simulink model "cruise_control_prop_error1"  (Simulink 7.8)
settings: Solver=FixedStepDiscrete  SolverMode=SingleTasking  StartTime=0.0  StopTime=50  FixedStep=0.01  RelTol=1e-3  AbsTol=1e-6
model workspace (MAT data in the model file):
  converter_data = [0  137.465208994  2.232; 0.1  137.065019157  2.075; 0.2  135.864449646  1.975; 0.3  135.664354728  1.846; 0.4  137.565256453  1.72; 0.5  140.366585312  1.564; 0.6  145.268910814  1.409; 0.7  152.872517717  1.254; 0.8  162.9773111  1.096; 0.81  164.27792807  1.08; 0.82  166.178829795  1.061; 0.83  167.979684062  1.043; 0.84  170.080680706  1.028; 0.85  172.781962105  1.012; 0.86  175.383196045  1.002; 0.87  179.585189333  1.002; 0.88  183.587087703  1.001; 0.89  189.890077635  0.998; 0.9  197.693779455  0.999; 0.92  215.902417037  1.001; 0.94  244.515990379  1.002]
  emap = [-40  -44  -49  -53  -57  -61  -65  -70  -74  -78  -82; 215  117  85  66  44  29  10  -2  -13  -22  -32; 245  208  178  148  122  104  85  66  48  33  18; 264  260  241  219  193  167  152  133  119  96  85; 264  279  282  275  260  238  223  208  189  171  152; 267  290  293  297  290  275  260  256  234  212  193; 267  297  305  305  305  301  293  282  267  249  226; 267  301  308  312  319  323  319  316  297  279  253; 267  301  312  319  327  327  327  327  312  293  267; 267  301  312  319  327  334  334  334  319  305  275]
  Iei = 0.0219914882836
  nevec = [800 1200 1600 2000 2400 2800 3200 3600 4000 4400 4800]
  p0 = 0.07934
  p1 = 0.07934
  thvec = [0; 20; 30; 40; 50; 60; 70; 80; 90; 100]
  vehicledata : num (value not decoded)
values from neighbouring files (symbols this model uses):
  cruise_ki = 0.01    [cruise_control_data.m]    (also in fxpdata_simulinkpackage.mat)
  cruise_kp = 0.02    [cruise_control_data.m]    (also in fxpdata_simulinkpackage.mat)
  speed_max = 300    [cruise_control_data.m]    (also in fxpdata_simulinkpackage.mat)
  speed_min = -50    [cruise_control_data.m]    (also in fxpdata_simulinkpackage.mat)
  target_max = 100    [cruise_control_data.m]    (also in fxpdata_simulinkpackage.mat)
  target_min = 30    [cruise_control_data.m]    (also in fxpdata_simulinkpackage.mat)
  throt_max = 100    [cruise_control_data.m]    (also in fxpdata_simulinkpackage.mat)
  throt_min = 0    [cruise_control_data.m]    (also in fxpdata_simulinkpackage.mat)
  vel_dec = 1    [cruise_control_data.m]    (also in fxpdata_simulinkpackage.mat)
  vel_inc = 1    [cruise_control_data.m]    (also in fxpdata_simulinkpackage.mat)
undefined symbols (not defined in the file or in its folder): DiscIntNeverNeededParam, sldvsubsys
libraries: sldvlib x29, propertySpecificationOperatorLib x8, simulink x1
settings Model: MinMaxOverflowLogging=MinMaxAndOverflow  FPTRunName=オーバーライドなし  Creator=The MathWorks Inc.  LastModifiedBy=itoy  CovMetricSettings=dcmtr  CovHTMLOptions=-aTS=1 -bRG=1 -bTC=1 -hTR=0 -nFC=0 -scm=1 -bcm=1 -xEv=0  ExtModeTrigMode=oneshot  ExtModeArmWhenConnect=off  ExtModeAutoUpdateStatusClock=off
settings DataIOCC: LimitDataPoints=off  SaveOutput=off  SaveTime=off  SignalLoggingName=mysig
settings OptimizationCC: InlineParams=on  UseIntDivNetSlope=on  UseFloatMulNetSlope=on  InlineInvariantSignals=on  EnhancedBackFolding=on  EfficientFloat2IntCast=on  LifeSpan=1
settings DebuggingCC: SignalInfNanChecking=error  SaveWithParameterizedLinksMsg=none  CheckExecutionContextPreStartOutputMsg=on  CheckExecutionContextRuntimeOutputMsg=on  SolverPrmCheckMsg=none  SingleTaskRateTransMsg=error  IntegerOverflowMsg=error  UniqueDataStoreMsg=error  BusObjectLabelMismatch=error  RootOutportRequireBusObject=error  AssertControl=DisableAll  StrictBusMsg=ErrorOnBusTreatedAsVector  BusNameAdapt=ErrorWithoutRepair  NonBusSignalsTreatedAsBus=error  LoggingUnavailableSignals=none
settings HardwareCC: ProdIntDivRoundTo=Zero  ProdEndianess=LittleEndian  ProdHWDeviceType=NEC->V850  TargetIntDivRoundTo=Zero  TargetEndianess=LittleEndian  TargetHWDeviceType=MATLAB Host
settings ModelReferenceCC: ModelReferenceNumInstancesAllowed=Single
settings SFSimCC: SFSimEcho=off  SimParseCustomCode=off
settings RTWCC: GenerateReport=on  ProcessScript=grt_make_rtw_hook  LaunchReport=on  IncludeERTFirstTime=on  RTWCompilerOptimization=On
settings ConfigComp: Description=Design Verifier Custom Configuration Component  DVMaxProcessTime=3000  DVDisplayUnsatisfiableObjectives=on  DVModelCoverageObjectives=MCDC  DVMaxTestCaseSteps=500  DVTestSuiteOptimization=LargeModel (Nonlinear Extended)

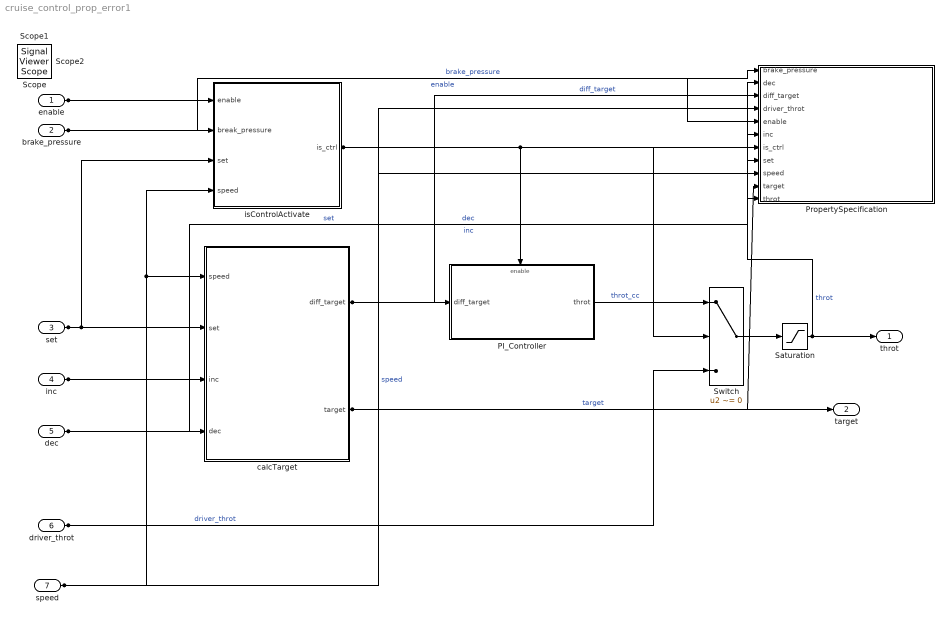
== system cruise_control_prop_error1 ==
  enable : Inport  PortDimensions=1  Interpolate=off
  brake_pressure : Inport  Port=2  PortDimensions=1  Interpolate=off
  set : Inport  Port=3  PortDimensions=1  Interpolate=off
  inc : Inport  Port=4  PortDimensions=1  Interpolate=off
  dec : Inport  Port=5  PortDimensions=1  Interpolate=off
  driver_throt : Inport  Port=6  PortDimensions=1  Interpolate=off
  speed : Inport  Port=7  PortDimensions=1  Interpolate=off
  PI_Controller : Subsystem
  PropertySpecification : Subsystem  Tag=VerificationSubsystem  DisableCoverage=on  LoadFcn=sldvsubsys('check')  TreatAsAtomicUnit=on  SimViewingDevice=on  mask(VerificationSubsystem){}
      mask help: aa
      mask init:
      | sldvsubsys('maskInit');
      settings: OpenFcn=PropertySpecificationUI('Block',gcb)
      settings: CopyFcn=|
      | sldvsubsys('copy');
      |  set_param(gcb,'LinkStatus','none')
      settings: PreSaveFcn=|
      | set_param(gcb,'SimViewingDevice','on');
      | sldvsubsys('check');
      mask Help: helpview(fullfile(docroot,'toolbox','sldv','sldv.map'),'verificationsubsystem')
      mask Display: image(imread('sldvicon_versubsys.png','BackGroundColor',[1 1 1]),'center');
  Saturation : Saturate  UpperLimit=throt_max  LowerLimit=throt_min  OutDataTypeStr=Inherit: Inherit via back propagation
      settings: AttributesFormatString=<UpperLimit = %<UpperLimit>>\n<LowerLimit = %<LowerLimit>>
  Switch : Switch  Criteria=u2 ~= 0  OutDataTypeStr=Inherit: Inherit via back propagation
      settings: AttributesFormatString=<Criteria=%<Criteria>>
  calcTarget : Subsystem
  isControlActivate : Subsystem
  throt : Outport  PortDimensions=[1 1]
  target : Outport  Port=2  PortDimensions=[1 1]
  Scope : SignalViewerScope  IOType=viewer  NumInputPorts=7  RefreshTime=0.035000
      settings: YMin=-5~-5~-5~-5~-5~-5~-5  YMax=5~5~5~5~5~5~5
  Scope1 : SignalViewerScope  IOType=viewer  NumInputPorts=3  RefreshTime=0.035000
      settings: YMin=-5~-5~-5  YMax=5~5~5
  Scope2 : SignalViewerScope  IOType=viewer  NumInputPorts=2  RefreshTime=0.035000
      settings: YMin=-5~-5  YMax=5~5  SaveName=ScopeData2
  wires:
  isControlActivate/1(is_ctrl) -> Switch/2, PI_Controller/Enable, PropertySpecification/7(is_ctrl)
  calcTarget/2(target) -> target/1, PropertySpecification/10(target)  "target"
  calcTarget/1(diff_target) -> PI_Controller/1(diff_target), PropertySpecification/3(diff_target)  "diff_target"
  dec/1 -> calcTarget/4(dec), PropertySpecification/2(dec)  "dec"
  speed/1 -> isControlActivate/4(speed), calcTarget/1(speed), PropertySpecification/9(speed)  "speed"
  inc/1 -> calcTarget/3(inc), PropertySpecification/6(inc)  "inc"
  set/1 -> isControlActivate/3(set), calcTarget/2(set), PropertySpecification/8(set)  "set"
  Switch/1 -> Saturation/1
  driver_throt/1 -> Switch/3, PropertySpecification/4(driver_throt)  "driver_throt"
  brake_pressure/1 -> isControlActivate/2(break_pressure), PropertySpecification/1(brake_pressure)  "brake_pressure"
  enable/1 -> isControlActivate/1(enable), PropertySpecification/5(enable)  "enable"
  PI_Controller/1(throt) -> Switch/1  "throt_cc"
  Saturation/1 -> throt/1, PropertySpecification/11(throt)  "throt"

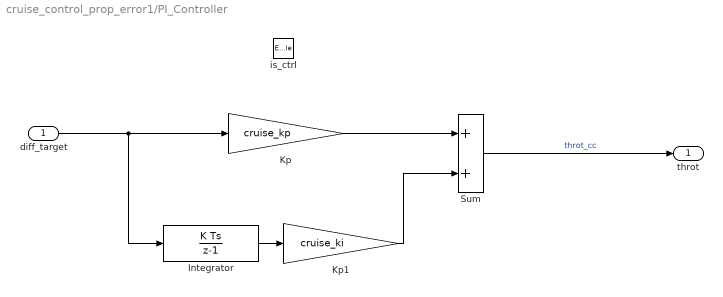
== system cruise_control_prop_error1/PI_Controller ==
  diff_target : Inport
  is_ctrl : EnablePort  StatesWhenEnabling=reset
  Integrator : DiscreteIntegrator  gainval=1  InitialConditionMode=State only (most efficient)  SampleTime=-1  UpperSaturationLimit=5  LowerSaturationLimit=-5  ICPrevOutput=DiscIntNeverNeededParam  ICPrevScaledInput=DiscIntNeverNeededParam
      settings: AttributesFormatString=<Gain = %<gainval>>\n<%<InitialConditionMode>>\n<SampleTime = %<SampleTime>>
  Kp : Gain  Gain=cruise_kp  ParamDataTypeStr=Inherit: Inherit from 'Gain'  OutDataTypeStr=Inherit: Inherit via back propagation
  Kp1 : Gain  Gain=cruise_ki  ParamDataTypeStr=Inherit: Inherit from 'Gain'  OutDataTypeStr=Inherit: Inherit via back propagation
  Sum : Sum  OutDataTypeStr=Inherit: Inherit via back propagation
  throt : Outport  InitialOutput=0
  wires:
  Kp1/1 -> Sum/2
  Kp/1 -> Sum/1
  Integrator/1 -> Kp1/1
  diff_target/1 -> Kp/1, Integrator/1
  Sum/1 -> throt/1  "throt_cc"

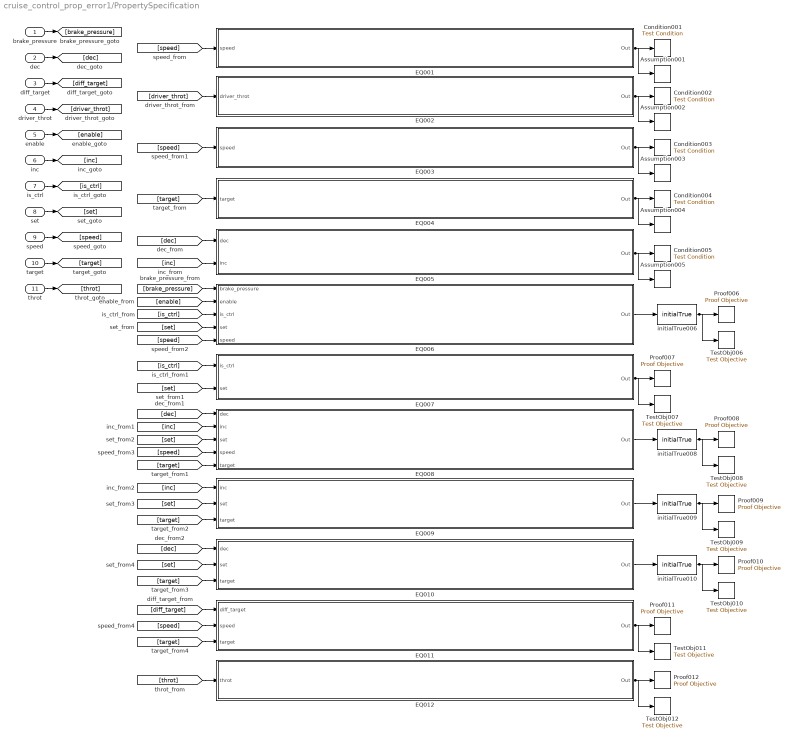
== system cruise_control_prop_error1/PropertySpecification ==
  brake_pressure : Inport
  dec : Inport  Port=2
  diff_target : Inport  Port=3
  driver_throt : Inport  Port=4
  enable : Inport  Port=5
  inc : Inport  Port=6
  is_ctrl : Inport  Port=7
  set : Inport  Port=8
  speed : Inport  Port=9
  target : Inport  Port=10
  throt : Inport  Port=11
  Assumption001 : sldvlib/Objectives and Constraints/Assumption  enabled=on  customAVTBlockType=Assumption  intervals=true  initial=off  dispValues=on  outEnabled=off
      settings: AttributesFormatString=%<intervals>
  Assumption002 : sldvlib/Objectives and Constraints/Assumption  enabled=on  customAVTBlockType=Assumption  intervals=true  initial=off  dispValues=on  outEnabled=off
      settings: AttributesFormatString=%<intervals>
  Assumption003 : sldvlib/Objectives and Constraints/Assumption  enabled=on  customAVTBlockType=Assumption  intervals=true  initial=off  dispValues=on  outEnabled=off
      settings: AttributesFormatString=%<intervals>
  Assumption004 : sldvlib/Objectives and Constraints/Assumption  enabled=on  customAVTBlockType=Assumption  intervals=true  initial=off  dispValues=on  outEnabled=off
      settings: AttributesFormatString=%<intervals>
  Assumption005 : sldvlib/Objectives and Constraints/Assumption  enabled=on  customAVTBlockType=Assumption  intervals=true  initial=off  dispValues=on  outEnabled=off
      settings: AttributesFormatString=%<intervals>
  Condition001 : sldvlib/Objectives and Constraints/Test Condition  enabled=on  customAVTBlockType=Test Condition  intervals=true  initial=off  dispValues=on  outEnabled=off
      settings: AttributesFormatString=%<intervals>
  Condition002 : sldvlib/Objectives and Constraints/Test Condition  enabled=on  customAVTBlockType=Test Condition  intervals=true  initial=off  dispValues=on  outEnabled=off
      settings: AttributesFormatString=%<intervals>
  Condition003 : sldvlib/Objectives and Constraints/Test Condition  enabled=on  customAVTBlockType=Test Condition  intervals=true  initial=off  dispValues=on  outEnabled=off
      settings: AttributesFormatString=%<intervals>
  Condition004 : sldvlib/Objectives and Constraints/Test Condition  enabled=on  customAVTBlockType=Test Condition  intervals=true  initial=off  dispValues=on  outEnabled=off
      settings: AttributesFormatString=%<intervals>
  Condition005 : sldvlib/Objectives and Constraints/Test Condition  enabled=on  customAVTBlockType=Test Condition  intervals=true  initial=off  dispValues=on  outEnabled=off
      settings: AttributesFormatString=%<intervals>
  EQ001 : Subsystem  Tag=CustomScope  mask(sldvLiteralTemporalLogicLib){InputVar=speed, ParamVar=speed_max,speed_min, VerifEq=speed_min <= speed && speed <= speed_max}
      mask prompts: InputVar "入力変数"; ParamVar "パラメータ変数"; VerifEq "検査式"
      mask help: sldvLiteralTemporalLogiclib
      mask init:
      | literalEq2SimulinkCallback(gcb,InputVar,ParamVar,VerifEq)
      mask Display: disp(VerifEq)
  EQ002 : Subsystem  Tag=CustomScope  mask(sldvLiteralTemporalLogicLib){InputVar=driver_throt, ParamVar=throt_max,throt_min, VerifEq=throt_min <= driver_throt && driver_throt <= throt_max}
      mask prompts: InputVar "入力変数"; ParamVar "パラメータ変数"; VerifEq "検査式"
      mask help: sldvLiteralTemporalLogiclib
      mask init:
      | literalEq2SimulinkCallback(gcb,InputVar,ParamVar,VerifEq)
      mask Display: disp(VerifEq)
  EQ003 : Subsystem  Tag=CustomScope  mask(sldvLiteralTemporalLogicLib){InputVar=speed, ParamVar=, VerifEq=init(speed==0,1)}
      mask prompts: InputVar "入力変数"; ParamVar "パラメータ変数"; VerifEq "検査式"
      mask help: sldvLiteralTemporalLogiclib
      mask init:
      | literalEq2SimulinkCallback(gcb,InputVar,ParamVar,VerifEq)
      mask Display: disp(VerifEq)
  EQ004 : Subsystem  Tag=CustomScope  mask(sldvLiteralTemporalLogicLib){InputVar=target, ParamVar=target_min, VerifEq=init(target==target_min,1)}
      mask prompts: InputVar "入力変数"; ParamVar "パラメータ変数"; VerifEq "検査式"
      mask help: sldvLiteralTemporalLogiclib
      mask init:
      | literalEq2SimulinkCallback(gcb,InputVar,ParamVar,VerifEq)
      mask Display: disp(VerifEq)
  EQ005 : Subsystem  Tag=CustomScope  mask(sldvLiteralTemporalLogicLib){InputVar=dec,inc, ParamVar=, VerifEq=~(inc && dec)}
      mask prompts: InputVar "入力変数"; ParamVar "パラメータ変数"; VerifEq "検査式"
      mask help: sldvLiteralTemporalLogiclib
      mask init:
      | literalEq2SimulinkCallback(gcb,InputVar,ParamVar,VerifEq)
      mask Display: disp(VerifEq)
  EQ006 : Subsystem  Tag=CustomScope  mask(sldvLiteralTemporalLogicLib){InputVar=brake_pressure,enable,is_ctrl,set,speed, ParamVar=target_max,target_min, VerifEq=enable && brake_pressure == 0 && ( set || prev(is_ctrl,1) ) && (target_min <= speed && speed <= target_max) ==> is_ctrl}
      mask prompts: InputVar "入力変数"; ParamVar "パラメータ変数"; VerifEq "検査式"
      mask help: sldvLiteralTemporalLogiclib
      mask init:
      | literalEq2SimulinkCallback(gcb,InputVar,ParamVar,VerifEq)
      mask Display: disp(VerifEq)
  EQ007 : Subsystem  Tag=CustomScope  mask(sldvLiteralTemporalLogicLib){InputVar=is_ctrl,set, ParamVar=, VerifEq=init(~set,1) ==> init(~is_ctrl,1)}
      mask prompts: InputVar "入力変数"; ParamVar "パラメータ変数"; VerifEq "検査式"
      mask help: sldvLiteralTemporalLogiclib
      mask init:
      | literalEq2SimulinkCallback(gcb,InputVar,ParamVar,VerifEq)
      mask Display: disp(VerifEq)
  EQ008 : Subsystem  Tag=CustomScope  mask(sldvLiteralTemporalLogicLib){InputVar=dec,inc,set,speed,target, ParamVar=target_max,target_min, VerifEq=set && (inc || dec) && (target_min <= speed && speed <= target_max) ==> target == speed}
      mask prompts: InputVar "入力変数"; ParamVar "パラメータ変数"; VerifEq "検査式"
      mask help: sldvLiteralTemporalLogiclib
      mask init:
      | literalEq2SimulinkCallback(gcb,InputVar,ParamVar,VerifEq)
      mask Display: disp(VerifEq)
  EQ009 : Subsystem  Tag=CustomScope  mask(sldvLiteralTemporalLogicLib){InputVar=inc,set,target, ParamVar=target_max,target_min,vel_inc, VerifEq=inc && (target_min < target && target < target_max) && ~set ==> (target - prev(target,1)) == vel_inc}
      mask prompts: InputVar "入力変数"; ParamVar "パラメータ変数"; VerifEq "検査式"
      mask help: sldvLiteralTemporalLogiclib
      mask init:
      | literalEq2SimulinkCallback(gcb,InputVar,ParamVar,VerifEq)
      mask Display: disp(VerifEq)
  EQ010 : Subsystem  Tag=CustomScope  mask(sldvLiteralTemporalLogicLib){InputVar=dec,set,target, ParamVar=target_max,target_min,vel_dec, VerifEq=dec && (target_min < target && target < target_max) && ~set ==> (target - prev(target,1)) == -vel_dec}
      mask prompts: InputVar "入力変数"; ParamVar "パラメータ変数"; VerifEq "検査式"
      mask help: sldvLiteralTemporalLogiclib
      mask init:
      | literalEq2SimulinkCallback(gcb,InputVar,ParamVar,VerifEq)
      mask Display: disp(VerifEq)
  EQ011 : Subsystem  Tag=CustomScope  mask(sldvLiteralTemporalLogicLib){InputVar=diff_target,speed,target, ParamVar=, VerifEq=diff_target == target - speed}
      mask prompts: InputVar "入力変数"; ParamVar "パラメータ変数"; VerifEq "検査式"
      mask help: sldvLiteralTemporalLogiclib
      mask init:
      | literalEq2SimulinkCallback(gcb,InputVar,ParamVar,VerifEq)
      mask Display: disp(VerifEq)
  EQ012 : Subsystem  Tag=CustomScope  mask(sldvLiteralTemporalLogicLib){InputVar=throt, ParamVar=throt_max,throt_min, VerifEq=~(throt_min > throt || throt > throt_max)}
      mask prompts: InputVar "入力変数"; ParamVar "パラメータ変数"; VerifEq "検査式"
      mask help: sldvLiteralTemporalLogiclib
      mask init:
      | literalEq2SimulinkCallback(gcb,InputVar,ParamVar,VerifEq)
      mask Display: disp(VerifEq)
  Proof006 : sldvlib/Objectives and Constraints/Proof Objective  enabled=on  customAVTBlockType=Proof Objective  intervals=true  dispValues=on  outEnabled=off  enableStopSim=off
      settings: AttributesFormatString=%<intervals>
  Proof007 : sldvlib/Objectives and Constraints/Proof Objective  enabled=on  customAVTBlockType=Proof Objective  intervals=true  dispValues=on  outEnabled=off  enableStopSim=off
      settings: AttributesFormatString=%<intervals>
  Proof008 : sldvlib/Objectives and Constraints/Proof Objective  enabled=on  customAVTBlockType=Proof Objective  intervals=true  dispValues=on  outEnabled=off  enableStopSim=off
      settings: AttributesFormatString=%<intervals>
  Proof009 : sldvlib/Objectives and Constraints/Proof Objective  enabled=on  customAVTBlockType=Proof Objective  intervals=true  dispValues=on  outEnabled=off  enableStopSim=off
      settings: AttributesFormatString=%<intervals>
  Proof010 : sldvlib/Objectives and Constraints/Proof Objective  enabled=on  customAVTBlockType=Proof Objective  intervals=true  dispValues=on  outEnabled=off  enableStopSim=off
      settings: AttributesFormatString=%<intervals>
  Proof011 : sldvlib/Objectives and Constraints/Proof Objective  enabled=on  customAVTBlockType=Proof Objective  intervals=true  dispValues=on  outEnabled=off  enableStopSim=off
      settings: AttributesFormatString=%<intervals>
  Proof012 : sldvlib/Objectives and Constraints/Proof Objective  enabled=on  customAVTBlockType=Proof Objective  intervals=true  dispValues=on  outEnabled=off  enableStopSim=off
      settings: AttributesFormatString=%<intervals>
  TestObj006 : sldvlib/Objectives and Constraints/Test Objective  enabled=off  customAVTBlockType=Test Objective  intervals=true  dispValues=on  outEnabled=off
      settings: AttributesFormatString=%<intervals>
  TestObj007 : sldvlib/Objectives and Constraints/Test Objective  enabled=off  customAVTBlockType=Test Objective  intervals=true  dispValues=on  outEnabled=off
      settings: AttributesFormatString=%<intervals>
  TestObj008 : sldvlib/Objectives and Constraints/Test Objective  enabled=off  customAVTBlockType=Test Objective  intervals=true  dispValues=on  outEnabled=off
      settings: AttributesFormatString=%<intervals>
  TestObj009 : sldvlib/Objectives and Constraints/Test Objective  enabled=off  customAVTBlockType=Test Objective  intervals=true  dispValues=on  outEnabled=off
      settings: AttributesFormatString=%<intervals>
  TestObj010 : sldvlib/Objectives and Constraints/Test Objective  enabled=off  customAVTBlockType=Test Objective  intervals=true  dispValues=on  outEnabled=off
      settings: AttributesFormatString=%<intervals>
  TestObj011 : sldvlib/Objectives and Constraints/Test Objective  enabled=off  customAVTBlockType=Test Objective  intervals=true  dispValues=on  outEnabled=off
      settings: AttributesFormatString=%<intervals>
  TestObj012 : sldvlib/Objectives and Constraints/Test Objective  enabled=off  customAVTBlockType=Test Objective  intervals=true  dispValues=on  outEnabled=off
      settings: AttributesFormatString=%<intervals>
  initialTrue006 : propertySpecificationOperatorLib/initialTrue  DelayCount=1
  initialTrue008 : propertySpecificationOperatorLib/initialTrue  DelayCount=1
  initialTrue009 : propertySpecificationOperatorLib/initialTrue  DelayCount=1
  initialTrue010 : propertySpecificationOperatorLib/initialTrue  DelayCount=1
  wires:
  brake_pressure/1 -> [brake_pressure]
  dec/1 -> [dec]
  diff_target/1 -> [diff_target]
  driver_throt/1 -> [driver_throt]
  enable/1 -> [enable]
  inc/1 -> [inc]
  is_ctrl/1 -> [is_ctrl]
  set/1 -> [set]
  speed/1 -> [speed]
  target/1 -> [target]
  throt/1 -> [throt]
  [speed] -> EQ001/1(speed)
  [driver_throt] -> EQ002/1(driver_throt)
  [speed] -> EQ003/1(speed)
  [target] -> EQ004/1(target)
  [dec] -> EQ005/1(dec)
  [inc] -> EQ005/2(inc)
  [brake_pressure] -> EQ006/1(brake_pressure)
  [enable] -> EQ006/2(enable)
  [is_ctrl] -> EQ006/3(is_ctrl)
  [set] -> EQ006/4(set)
  [speed] -> EQ006/5(speed)
  [is_ctrl] -> EQ007/1(is_ctrl)
  [set] -> EQ007/2(set)
  [dec] -> EQ008/1(dec)
  [inc] -> EQ008/2(inc)
  [set] -> EQ008/3(set)
  [speed] -> EQ008/4(speed)
  [target] -> EQ008/5(target)
  [inc] -> EQ009/1(inc)
  [set] -> EQ009/2(set)
  [target] -> EQ009/3(target)
  [dec] -> EQ010/1(dec)
  [set] -> EQ010/2(set)
  [target] -> EQ010/3(target)
  [diff_target] -> EQ011/1(diff_target)
  [speed] -> EQ011/2(speed)
  [target] -> EQ011/3(target)
  [throt] -> EQ012/1(throt)
  EQ001/1(Out) -> Condition001/1, Assumption001/1
  EQ002/1(Out) -> Condition002/1, Assumption002/1
  EQ003/1(Out) -> Condition003/1, Assumption003/1
  EQ004/1(Out) -> Condition004/1, Assumption004/1
  EQ005/1(Out) -> Condition005/1, Assumption005/1
  initialTrue006/1 -> Proof006/1, TestObj006/1
  EQ007/1(Out) -> Proof007/1, TestObj007/1
  initialTrue008/1 -> Proof008/1, TestObj008/1
  initialTrue009/1 -> Proof009/1, TestObj009/1
  initialTrue010/1 -> Proof010/1, TestObj010/1
  EQ011/1(Out) -> Proof011/1, TestObj011/1
  EQ012/1(Out) -> Proof012/1, TestObj012/1
  EQ006/1(Out) -> initialTrue006/1
  EQ008/1(Out) -> initialTrue008/1
  EQ009/1(Out) -> initialTrue009/1
  EQ010/1(Out) -> initialTrue010/1

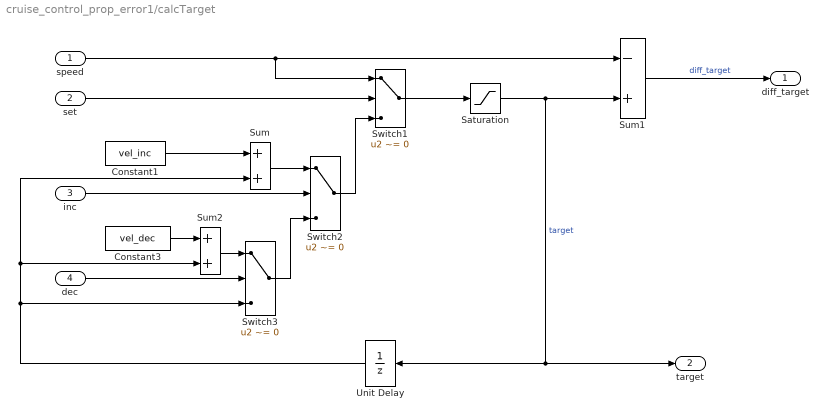
== system cruise_control_prop_error1/calcTarget ==
  speed : Inport
  set : Inport  Port=2
  inc : Inport  Port=3
  dec : Inport  Port=4
  Constant1 : Constant  Value=vel_inc  OutDataTypeStr=Inherit: Inherit via back propagation
  Constant3 : Constant  Value=vel_dec  OutDataTypeStr=Inherit: Inherit via back propagation
  Saturation : Saturate  UpperLimit=target_max  LowerLimit=target_min
      settings: AttributesFormatString=<UpperLimit = %<UpperLimit>>\n<LowerLimit = %<LowerLimit>>
  Sum : Sum
  Sum1 : Sum  Inputs=-+  OutDataTypeStr=Inherit: Same as first input
  Sum2 : Sum
  Switch1 : Switch  Criteria=u2 ~= 0
      settings: AttributesFormatString=<Criteria=%<Criteria>>
  Switch2 : Switch  Criteria=u2 ~= 0
      settings: AttributesFormatString=<Criteria=%<Criteria>>
  Switch3 : Switch  Criteria=u2 ~= 0
      settings: AttributesFormatString=<Criteria=%<Criteria>>
  Unit Delay : UnitDelay  SampleTime=-1
      settings: AttributesFormatString=<InitValue = %<X0>>
  diff_target : Outport
  target : Outport  Port=2
  wires:
  Saturation/1 -> Sum1/2, target/1, Unit Delay/1  "target"
  set/1 -> Switch1/2
  speed/1 -> Switch1/1, Sum1/1
  inc/1 -> Switch2/2
  Constant1/1 -> Sum/1
  Sum/1 -> Switch2/1
  dec/1 -> Switch3/2
  Constant3/1 -> Sum2/1
  Sum2/1 -> Switch3/1
  Switch2/1 -> Switch1/3
  Switch3/1 -> Switch2/3
  Unit Delay/1 -> Switch3/3, Sum2/2, Sum/2
  Switch1/1 -> Saturation/1
  Sum1/1 -> diff_target/1  "diff_target"

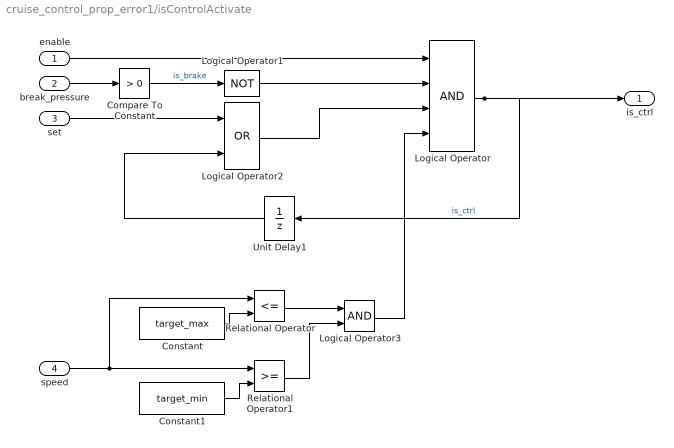
== system cruise_control_prop_error1/isControlActivate ==
  enable : Inport
  break_pressure : Inport  Port=2
  set : Inport  Port=3
  speed : Inport  Port=4
  Compare To Constant : simulink/Logic and Bit Operations/Compare To Constant  relop=>  const=0  OutDataTypeStr=boolean
  Constant : Constant  Value=target_max
  Constant1 : Constant  Value=target_min
  Logical Operator : Logic  Inputs=4  AllPortsSameDT=off  OutDataTypeStr=boolean
  Logical Operator1 : Logic  Operator=NOT  AllPortsSameDT=off  OutDataTypeStr=boolean
  Logical Operator2 : Logic  Operator=OR  AllPortsSameDT=off  OutDataTypeStr=boolean
  Logical Operator3 : Logic  AllPortsSameDT=off  OutDataTypeStr=boolean
  Relational Operator : RelationalOperator  Operator=<=  OutDataTypeStr=boolean
  Relational Operator1 : RelationalOperator  OutDataTypeStr=boolean
  Unit Delay1 : UnitDelay  X0=1  SampleTime=-1
      settings: AttributesFormatString=<InitValue = %<X0>>
  is_ctrl : Outport
  wires:
  Compare To Constant/1 -> Logical Operator1/1  "is_brake"
  Constant/1 -> Relational Operator/2
  Logical Operator3/1 -> Logical Operator/4
  Relational Operator1/1 -> Logical Operator3/2
  Relational Operator/1 -> Logical Operator3/1
  speed/1 -> Relational Operator/1, Relational Operator1/1
  Constant1/1 -> Relational Operator1/2
  break_pressure/1 -> Compare To Constant/1
  enable/1 -> Logical Operator/1
  set/1 -> Logical Operator2/1
  Logical Operator1/1 -> Logical Operator/2
  Logical Operator2/1 -> Logical Operator/3
  Unit Delay1/1 -> Logical Operator2/2
  Logical Operator/1 -> is_ctrl/1, Unit Delay1/1  "is_ctrl"

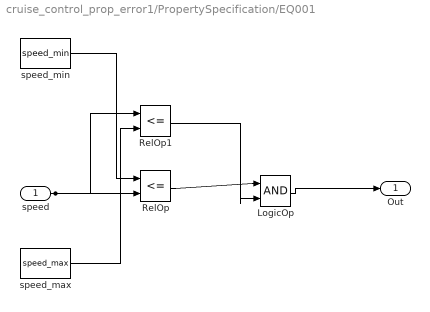
== system cruise_control_prop_error1/PropertySpecification/EQ001 ==
  speed : Inport
  LogicOp : Logic  AllPortsSameDT=off  OutDataTypeStr=boolean
  RelOp : RelationalOperator  Operator=<=  OutDataTypeStr=boolean
  RelOp1 : RelationalOperator  Operator=<=  OutDataTypeStr=boolean
  speed_max : Constant  Value=speed_max
  speed_min : Constant  Value=speed_min
  Out : Outport
  wires:
  RelOp/1 -> LogicOp/1
  speed/1 -> RelOp/2, RelOp1/1
  LogicOp/1 -> Out/1
  RelOp1/1 -> LogicOp/2
  speed_min/1 -> RelOp/1
  speed_max/1 -> RelOp1/2

== system cruise_control_prop_error1/PropertySpecification/EQ002 ==
  driver_throt : Inport
  LogicOp : Logic  AllPortsSameDT=off  OutDataTypeStr=boolean
  RelOp : RelationalOperator  Operator=<=  OutDataTypeStr=boolean
  RelOp1 : RelationalOperator  Operator=<=  OutDataTypeStr=boolean
  throt_max : Constant  Value=throt_max
  throt_min : Constant  Value=throt_min
  Out : Outport
  wires:
  RelOp/1 -> LogicOp/1
  driver_throt/1 -> RelOp/2, RelOp1/1
  LogicOp/1 -> Out/1
  RelOp1/1 -> LogicOp/2
  throt_min/1 -> RelOp/1
  throt_max/1 -> RelOp1/2

== system cruise_control_prop_error1/PropertySpecification/EQ003 ==
  speed : Inport
  Constant : Constant  Value=0  OutDataTypeStr=Inherit: Inherit via back propagation
  RelOp : RelationalOperator  Operator===  OutDataTypeStr=boolean
  initialCondition : propertySpecificationOperatorLib/initialCondition  DelayCount=1
  Out : Outport
  wires:
  initialCondition/1 -> Out/1
  speed/1 -> RelOp/1
  RelOp/1 -> initialCondition/1
  Constant/1 -> RelOp/2

== system cruise_control_prop_error1/PropertySpecification/EQ004 ==
  target : Inport
  RelOp : RelationalOperator  Operator===  OutDataTypeStr=boolean
  initialCondition : propertySpecificationOperatorLib/initialCondition  DelayCount=1
  target_min : Constant  Value=target_min
  Out : Outport
  wires:
  initialCondition/1 -> Out/1
  target/1 -> RelOp/1
  RelOp/1 -> initialCondition/1
  target_min/1 -> RelOp/2

== system cruise_control_prop_error1/PropertySpecification/EQ005 ==
  dec : Inport
  inc : Inport  Port=2
  LogicOp : Logic  Operator=NOT  AllPortsSameDT=off  OutDataTypeStr=boolean
  LogicOp1 : Logic  AllPortsSameDT=off  OutDataTypeStr=boolean
  Out : Outport
  wires:
  LogicOp1/1 -> LogicOp/1
  inc/1 -> LogicOp1/1
  LogicOp/1 -> Out/1
  dec/1 -> LogicOp1/2

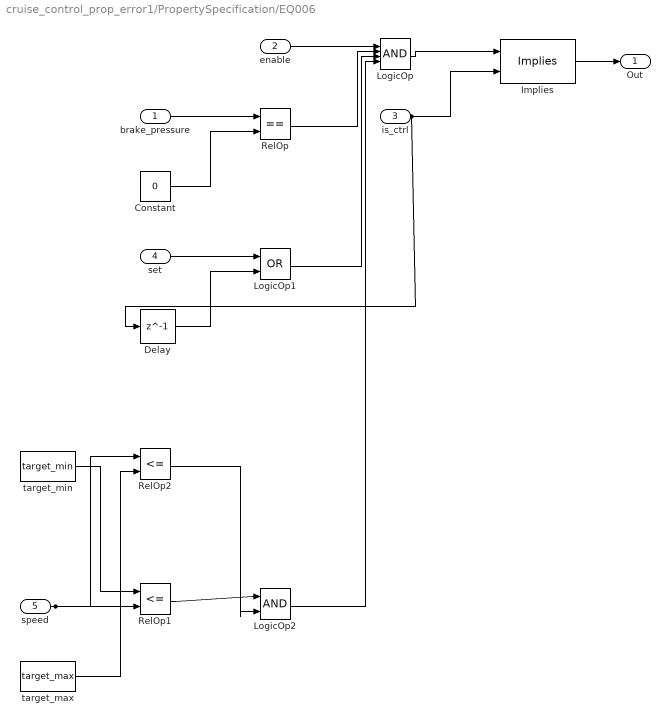
== system cruise_control_prop_error1/PropertySpecification/EQ006 ==
  brake_pressure : Inport
  enable : Inport  Port=2
  is_ctrl : Inport  Port=3
  set : Inport  Port=4
  speed : Inport  Port=5
  Constant : Constant  Value=0  OutDataTypeStr=Inherit: Inherit via back propagation
  Delay : Delay  DelayLength=1
  Implies : sldvlib/Verification Utilities/Implies
  LogicOp : Logic  Inputs=4  AllPortsSameDT=off  OutDataTypeStr=boolean
  LogicOp1 : Logic  Operator=OR  AllPortsSameDT=off  OutDataTypeStr=boolean
  LogicOp2 : Logic  AllPortsSameDT=off  OutDataTypeStr=boolean
  RelOp : RelationalOperator  Operator===  OutDataTypeStr=boolean
  RelOp1 : RelationalOperator  Operator=<=  OutDataTypeStr=boolean
  RelOp2 : RelationalOperator  Operator=<=  OutDataTypeStr=boolean
  target_max : Constant  Value=target_max
  target_min : Constant  Value=target_min
  Out : Outport
  wires:
  Implies/1 -> Out/1
  LogicOp/1 -> Implies/1
  enable/1 -> LogicOp/1
  set/1 -> LogicOp1/1
  RelOp1/1 -> LogicOp2/1
  brake_pressure/1 -> RelOp/1
  speed/1 -> RelOp1/2, RelOp2/1
  is_ctrl/1 -> Implies/2, Delay/1
  Delay/1 -> LogicOp1/2
  Constant/1 -> RelOp/2
  RelOp/1 -> LogicOp/2
  target_min/1 -> RelOp1/1
  RelOp2/1 -> LogicOp2/2
  target_max/1 -> RelOp2/2
  LogicOp1/1 -> LogicOp/3
  LogicOp2/1 -> LogicOp/4

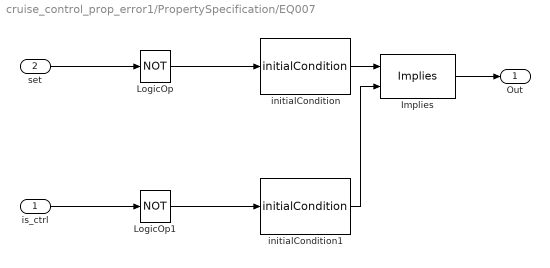
== system cruise_control_prop_error1/PropertySpecification/EQ007 ==
  is_ctrl : Inport
  set : Inport  Port=2
  Implies : sldvlib/Verification Utilities/Implies
  LogicOp : Logic  Operator=NOT  AllPortsSameDT=off  OutDataTypeStr=boolean
  LogicOp1 : Logic  Operator=NOT  AllPortsSameDT=off  OutDataTypeStr=boolean
  initialCondition : propertySpecificationOperatorLib/initialCondition  DelayCount=1
  initialCondition1 : propertySpecificationOperatorLib/initialCondition  DelayCount=1
  Out : Outport
  wires:
  initialCondition/1 -> Implies/1
  Implies/1 -> Out/1
  set/1 -> LogicOp/1
  is_ctrl/1 -> LogicOp1/1
  LogicOp/1 -> initialCondition/1
  LogicOp1/1 -> initialCondition1/1
  initialCondition1/1 -> Implies/2

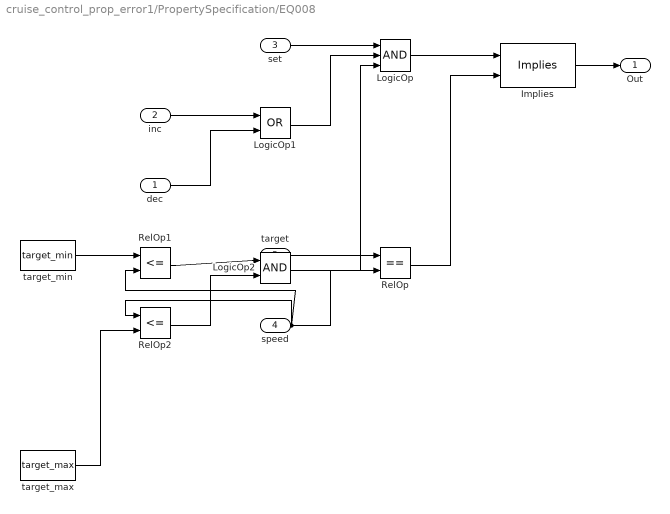
== system cruise_control_prop_error1/PropertySpecification/EQ008 ==
  dec : Inport
  inc : Inport  Port=2
  set : Inport  Port=3
  speed : Inport  Port=4
  target : Inport  Port=5
  Implies : sldvlib/Verification Utilities/Implies
  LogicOp : Logic  Inputs=3  AllPortsSameDT=off  OutDataTypeStr=boolean
  LogicOp1 : Logic  Operator=OR  AllPortsSameDT=off  OutDataTypeStr=boolean
  LogicOp2 : Logic  AllPortsSameDT=off  OutDataTypeStr=boolean
  RelOp : RelationalOperator  Operator===  OutDataTypeStr=boolean
  RelOp1 : RelationalOperator  Operator=<=  OutDataTypeStr=boolean
  RelOp2 : RelationalOperator  Operator=<=  OutDataTypeStr=boolean
  target_max : Constant  Value=target_max
  target_min : Constant  Value=target_min
  Out : Outport
  wires:
  Implies/1 -> Out/1
  target_min/1 -> RelOp1/1
  LogicOp/1 -> Implies/1
  set/1 -> LogicOp/1
  inc/1 -> LogicOp1/1
  RelOp1/1 -> LogicOp2/1
  target/1 -> RelOp/1
  RelOp2/1 -> LogicOp2/2
  dec/1 -> LogicOp1/2
  speed/1 -> RelOp/2, RelOp2/1, RelOp1/2
  LogicOp1/1 -> LogicOp/2
  target_max/1 -> RelOp2/2
  RelOp/1 -> Implies/2
  LogicOp2/1 -> LogicOp/3

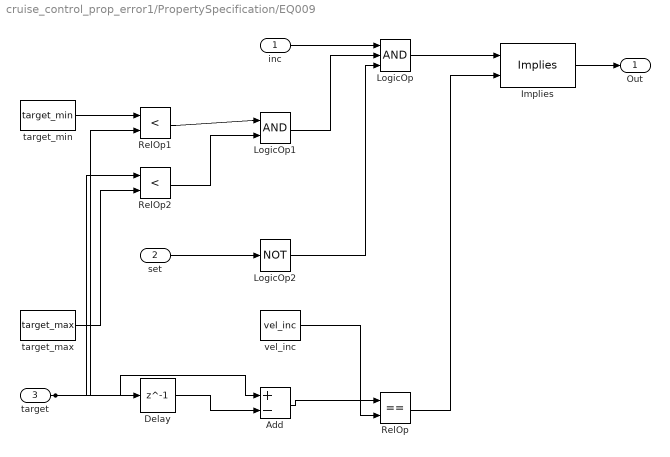
== system cruise_control_prop_error1/PropertySpecification/EQ009 ==
  inc : Inport
  set : Inport  Port=2
  target : Inport  Port=3
  Add : Sum  Inputs=+-
  Delay : Delay  DelayLength=1
  Implies : sldvlib/Verification Utilities/Implies
  LogicOp : Logic  Inputs=3  AllPortsSameDT=off  OutDataTypeStr=boolean
  LogicOp1 : Logic  AllPortsSameDT=off  OutDataTypeStr=boolean
  LogicOp2 : Logic  Operator=NOT  AllPortsSameDT=off  OutDataTypeStr=boolean
  RelOp : RelationalOperator  Operator===  OutDataTypeStr=boolean
  RelOp1 : RelationalOperator  Operator=<  OutDataTypeStr=boolean
  RelOp2 : RelationalOperator  Operator=<  OutDataTypeStr=boolean
  target_max : Constant  Value=target_max
  target_min : Constant  Value=target_min
  vel_inc : Constant  Value=vel_inc
  Out : Outport
  wires:
  Implies/1 -> Out/1
  target_min/1 -> RelOp1/1
  Delay/1 -> Add/2
  target/1 -> Delay/1, Add/1, RelOp2/1, RelOp1/2
  LogicOp/1 -> Implies/1
  inc/1 -> LogicOp/1
  RelOp1/1 -> LogicOp1/1
  set/1 -> LogicOp2/1
  Add/1 -> RelOp/1
  RelOp2/1 -> LogicOp1/2
  LogicOp1/1 -> LogicOp/2
  vel_inc/1 -> RelOp/2
  target_max/1 -> RelOp2/2
  LogicOp2/1 -> LogicOp/3
  RelOp/1 -> Implies/2

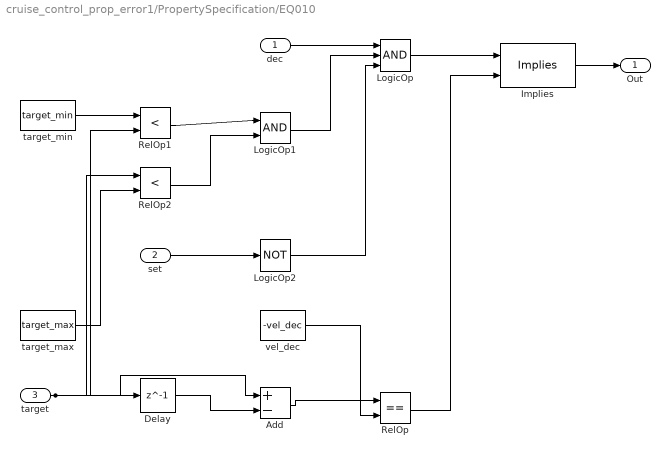
== system cruise_control_prop_error1/PropertySpecification/EQ010 ==
  dec : Inport
  set : Inport  Port=2
  target : Inport  Port=3
  Add : Sum  Inputs=+-
  Delay : Delay  DelayLength=1
  Implies : sldvlib/Verification Utilities/Implies
  LogicOp : Logic  Inputs=3  AllPortsSameDT=off  OutDataTypeStr=boolean
  LogicOp1 : Logic  AllPortsSameDT=off  OutDataTypeStr=boolean
  LogicOp2 : Logic  Operator=NOT  AllPortsSameDT=off  OutDataTypeStr=boolean
  RelOp : RelationalOperator  Operator===  OutDataTypeStr=boolean
  RelOp1 : RelationalOperator  Operator=<  OutDataTypeStr=boolean
  RelOp2 : RelationalOperator  Operator=<  OutDataTypeStr=boolean
  target_max : Constant  Value=target_max
  target_min : Constant  Value=target_min
  vel_dec : Constant  Value=-vel_dec
  Out : Outport
  wires:
  Implies/1 -> Out/1
  target_min/1 -> RelOp1/1
  Delay/1 -> Add/2
  target/1 -> Delay/1, Add/1, RelOp2/1, RelOp1/2
  LogicOp/1 -> Implies/1
  dec/1 -> LogicOp/1
  RelOp1/1 -> LogicOp1/1
  set/1 -> LogicOp2/1
  Add/1 -> RelOp/1
  RelOp2/1 -> LogicOp1/2
  LogicOp1/1 -> LogicOp/2
  vel_dec/1 -> RelOp/2
  target_max/1 -> RelOp2/2
  LogicOp2/1 -> LogicOp/3
  RelOp/1 -> Implies/2

== system cruise_control_prop_error1/PropertySpecification/EQ011 ==
  diff_target : Inport
  speed : Inport  Port=2
  target : Inport  Port=3
  Add : Sum  Inputs=+-
  RelOp : RelationalOperator  Operator===  OutDataTypeStr=boolean
  Out : Outport
  wires:
  target/1 -> Add/1
  diff_target/1 -> RelOp/1
  RelOp/1 -> Out/1
  speed/1 -> Add/2
  Add/1 -> RelOp/2

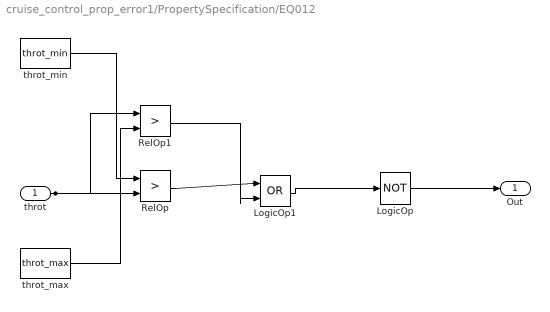
== system cruise_control_prop_error1/PropertySpecification/EQ012 ==
  throt : Inport
  LogicOp : Logic  Operator=NOT  AllPortsSameDT=off  OutDataTypeStr=boolean
  LogicOp1 : Logic  Operator=OR  AllPortsSameDT=off  OutDataTypeStr=boolean
  RelOp : RelationalOperator  Operator=>  OutDataTypeStr=boolean
  RelOp1 : RelationalOperator  Operator=>  OutDataTypeStr=boolean
  throt_max : Constant  Value=throt_max
  throt_min : Constant  Value=throt_min
  Out : Outport
  wires:
  LogicOp1/1 -> LogicOp/1
  RelOp/1 -> LogicOp1/1
  throt/1 -> RelOp/2, RelOp1/1
  LogicOp/1 -> Out/1
  RelOp1/1 -> LogicOp1/2
  throt_min/1 -> RelOp/1
  throt_max/1 -> RelOp1/2
